simulink model "partOneUnicycleRobot"  (R2021b)
settings: Solver=VariableStepAuto  StartTime=0.0  StopTime=10.0  RelTol=1e-3
settings Model: Creator=ericp  LastModifiedBy=ericp

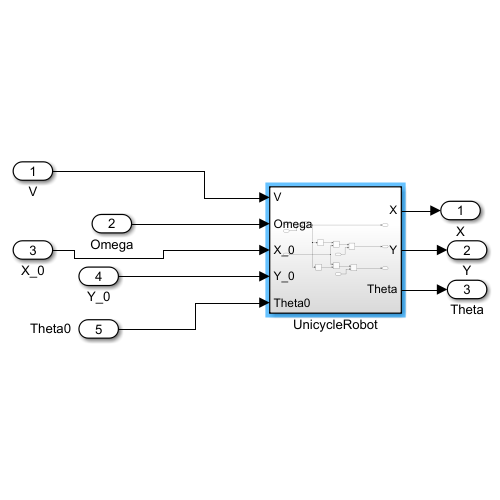
[thumbnail: Simulink's stored preview of the top-level diagram]
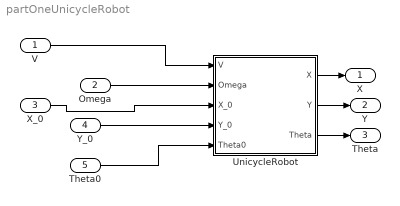
== system partOneUnicycleRobot ==
  V : Inport
  Omega : Inport  Port=2
  X_0 : Inport  Port=3
  Y_0 : Inport  Port=4
  Theta0 : Inport  Port=5
  UnicycleRobot : Subsystem
  X : Outport
  Y : Outport  Port=2
  Theta : Outport  Port=3
  wires:
  V/1 -> UnicycleRobot/1(V)
  Omega/1 -> UnicycleRobot/2(Omega)
  X_0/1 -> UnicycleRobot/3(X_0)
  Y_0/1 -> UnicycleRobot/4(Y_0)
  Theta0/1 -> UnicycleRobot/5(Theta0)
  UnicycleRobot/1(X) -> X/1
  UnicycleRobot/2(Y) -> Y/1
  UnicycleRobot/3(Theta) -> Theta/1

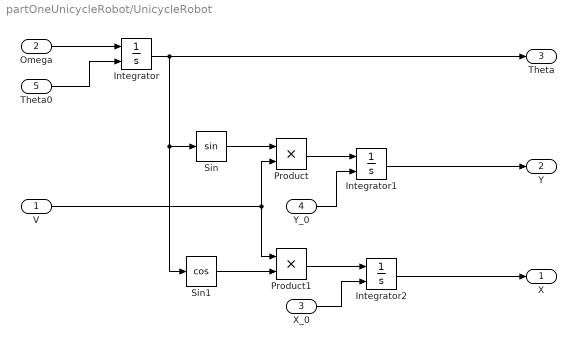
== system partOneUnicycleRobot/UnicycleRobot ==
  V : Inport
  Omega : Inport  Port=2
  X_0 : Inport  Port=3
  Y_0 : Inport  Port=4
  Theta0 : Inport  Port=5
  Integrator : Integrator  InitialConditionSource=external
  Integrator1 : Integrator  InitialConditionSource=external
  Integrator2 : Integrator  InitialConditionSource=external
  Product : Product
  Product1 : Product
  Sin : Trigonometry
  Sin1 : Trigonometry  Operator=cos
  X : Outport
  Y : Outport  Port=2
  Theta : Outport  Port=3
  wires:
  Sin1/1 -> Product1/2
  V/1 -> Product1/1, Product/2
  Integrator/1 -> Theta/1, Sin1/1, Sin/1
  Integrator2/1 -> X/1
  Sin/1 -> Product/1
  Theta0/1 -> Integrator/2
  Y_0/1 -> Integrator1/2
  Omega/1 -> Integrator/1
  X_0/1 -> Integrator2/2
  Integrator1/1 -> Y/1
  Product1/1 -> Integrator2/1
  Product/1 -> Integrator1/1
